simulink model "lab2_sinusoidal_input_2019b"  (R2022a)
settings: Solver=FixedStepAuto  StartTime=0.0  StopTime=70  RelTol=1e-3  EnableMultiTasking=on
undefined symbols (not defined in the file or in its folder): DiscIntNeverNeededParam
libraries: arduinolib x4
settings Model: ExtModeTrigDuration=2  Creator=MSI  LastModifiedBy=Owner
settings SolverCC: AlgebraicLoopSolver=TrustRegion
settings OptimizationCC: EnhancedBackFolding=on  PassReuseOutputArgsThreshold=0  MaxStackSize=64  OptimizeBlockOrder=speed  DifferentSizesBufferReuse=on  OptimizationCustomize=off
settings DebuggingCC: ParameterTunabilityLossMsg=error  UnconnectedInputMsg=warning  UnconnectedOutputMsg=warning  UnconnectedLineMsg=warning  SFMachineParentedDataDiag=warning
settings HardwareCC: ProdBitPerInt=16  ProdBitPerPointer=16  ProdBitPerSizeT=16  ProdBitPerPtrDiffT=16  ProdLargestAtomicFloat=None  ProdWordSize=8  ProdHWDeviceType=Atmel->AVR  UseEmbeddedCoderFeatures=off
settings SFSimCC: MATLABDynamicMemAlloc=off
settings RTWCC: SystemTargetFile=ert.tlc  HardwareBoard=Arduino Uno  TemplateMakefile=ert_default_tmf  GenerateReport=on  Toolchain=Arduino AVR  BuildConfiguration=Faster Runs  LaunchReport=on
settings CodeAppCC: ForceParamTrailComments=on  OperatorAnnotations=on
settings ERTTargetCC: ERTCustomFileBanners=off  SupportContinuousTime=on  SupportNonInlinedSFcns=on  RemoveResetFunc=off  SupportVariableSizeSignals=on  ModelStepFunctionPrototypeControlCompliant=off  ExtModeStaticAllocSize=250

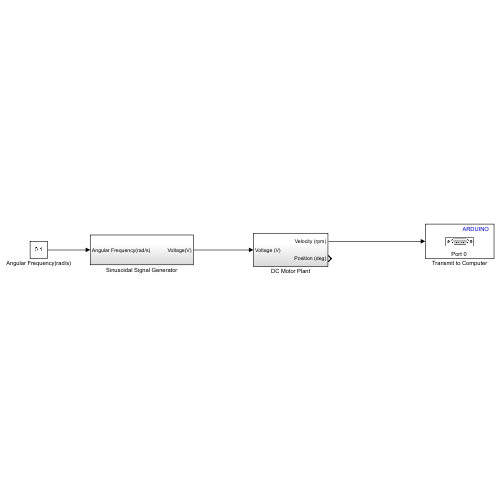
[thumbnail: Simulink's stored preview of the top-level diagram]
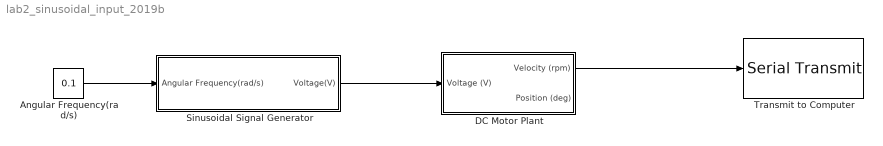
== system lab2_sinusoidal_input_2019b ==
  Angular Frequency(rad/s) : Constant  Value=0.1
  DC Motor Plant : Subsystem
  Sinusoidal Signal Generator : Subsystem
  Transmit to Computer : arduinolib/Serial Transmit  portNumber=0  sendmode=write  sendformat=Decimal  floatprecision=2  blockPlatform=arduino
  wires:
  DC Motor Plant/1(Velocity (rpm)) -> Transmit to Computer/1
  Angular Frequency(rad/s)/1 -> Sinusoidal Signal Generator/1(Angular Frequency(rad/s))
  Sinusoidal Signal Generator/1(Voltage(V)) -> DC Motor Plant/1(Voltage (V))

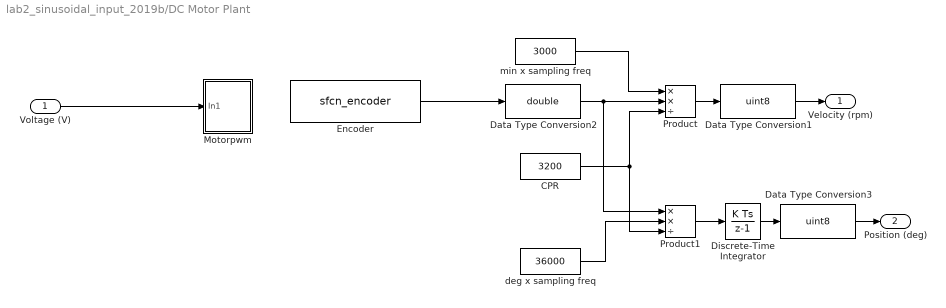
== system lab2_sinusoidal_input_2019b/DC Motor Plant ==
  Voltage (V) : Inport
  CPR : Constant  Value=3200
  Data Type Conversion1 : DataTypeConversion  OutDataTypeStr=uint8  SaturateOnIntegerOverflow=off  RndMeth=Floor
  Data Type Conversion2 : DataTypeConversion  OutDataTypeStr=double  RndMeth=Round  SaturateOnIntegerOverflow=off
  Data Type Conversion3 : DataTypeConversion  OutDataTypeStr=uint8  SaturateOnIntegerOverflow=off  RndMeth=Floor
  Discrete-Time Integrator : DiscreteIntegrator  SampleTime=-1  ICPrevOutput=DiscIntNeverNeededParam  ICPrevScaledInput=DiscIntNeverNeededParam
  Encoder : S-Function  InitFcn=try, set_param(gcb,'FunctionName','sfcn_encoder'), end  FunctionName=sfcn_encoder  Parameters=uint8(0),uint8(2),uint8(3)  SFunctionModules=sfcn_encoder_wrapper  SFunctionDeploymentMode=off  EnableBusSupport=off  mask(S-Function Builder){}
      mask init:
      | val = [[.9  0.75 0.75 1 1 .9 .9 1]',[1 1 0.75 0.75 .9 .9 1 .9]'];try , sys = get_param(gcb,'SfunBuilderFcnName');if isempty(sys), sys = get_param(gcb,'FunctionName'); end,catch, sys = get_param(gcb,'FunctionName'); end
      settings: CopyFcn=set_param(gcbh,'LinkStatus','none')  PreSaveFcn=try, set_param(gcb,'FunctionName','sfcn_encoder'), end  OpenFcn=sfunctionwizard(gcbh)
      mask Display: plot(val(:,1),val(:,2)),disp(sys), port_label('output',1,'pos')
  Motorpwm : Subsystem
  Product : Product  Inputs=**/
  Product1 : Product  Inputs=**/
  deg x sampling freq : Constant  Value=36000
  min x sampling freq : Constant  Value=3000
  Velocity (rpm) : Outport  VectorParamsAs1DForOutWhenUnconnected=off
  Position (deg) : Outport  Port=2  VectorParamsAs1DForOutWhenUnconnected=off
  wires:
  Voltage (V)/1 -> Motorpwm/1(In1)
  Data Type Conversion1/1 -> Velocity (rpm)/1
  Data Type Conversion2/1 -> Product1/1, Product/2
  CPR/1 -> Product1/3, Product/3
  Encoder/1 -> Data Type Conversion2/1
  Product1/1 -> Discrete-Time Integrator/1
  min x sampling freq/1 -> Product/1
  deg x sampling freq/1 -> Product1/2
  Product/1 -> Data Type Conversion1/1
  Data Type Conversion3/1 -> Position (deg)/1
  Discrete-Time Integrator/1 -> Data Type Conversion3/1

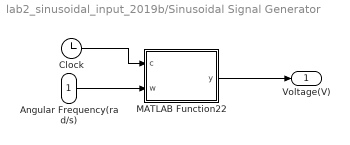
== system lab2_sinusoidal_input_2019b/Sinusoidal Signal Generator ==
  Angular Frequency(rad/s) : Inport
  Clock : Clock
  MATLAB Function22 : MATLAB Function  TreatAsAtomicUnit=on
  Voltage(V) : Outport
  wires:
  Clock/1 -> MATLAB Function22/1(c)
  MATLAB Function22/1(y) -> Voltage(V)/1
  Angular Frequency(rad/s)/1 -> MATLAB Function22/2(w)

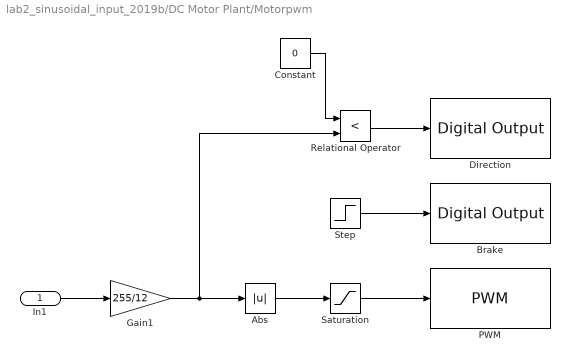
== system lab2_sinusoidal_input_2019b/DC Motor Plant/Motorpwm ==
  In1 : Inport
  Abs : Abs  SaturateOnIntegerOverflow=off
  Brake : arduinolib/Digital Output  pinNumber=8  Direction=output  blockPlatform=arduino
  Constant : Constant  Value=0
  "Direction " : arduinolib/Digital Output  pinNumber=13  Direction=output  blockPlatform=arduino
  Gain1 : Gain  Gain=255/12
  PWM : arduinolib/PWM  pinNumber=11  frequencyType=Default  desiredFrequency=490.2  achievableFrequency=490.2
  Relational Operator : RelationalOperator  Operator=<  OutDataTypeStr=boolean  RndMeth=Simplest  InputSameDT=off
  Saturation : Saturate  UpperLimit=255  LowerLimit=0
  Step : Step  Time=0  After=0  SampleTime=0
  wires:
  Relational Operator/1 -> "Direction "/1
  Step/1 -> Brake/1
  Saturation/1 -> PWM/1
  In1/1 -> Gain1/1
  Abs/1 -> Saturation/1
  Constant/1 -> Relational Operator/1
  Gain1/1 -> Relational Operator/2, Abs/1

== matlab function lab2_sinusoidal_input_2019b/Sinusoidal Signal Generator/MATLAB Function22 ==
  data: y output; c input; w input
function y = fcn2(c,w)
%#codegen
if w<1
    scale=70;
elseif w<10
    scale=25;
else
    scale=10;
end   
 
if c<scale
    y = 10*sin(w*c);
else
    y=0;
end
